simulink model "iterateddes"  (R2024b)
settings: Solver=VariableStepAuto  StartTime=0.0  StopTime=5  RelTol=1e-3
undefined symbols (not defined in the file or in its folder): entity, m, n, recordQueueTimeEng1, recordQueueTimeSrEng1, recordQueueTimeSrEng2, recordQueueTimeSrEng3, recordTotalTimeAdmin, recordTotalTimeInc, recordTotalTimeMaint, recordTotalTimeProj, recordTotalTimeReq
settings Model: Creator=enos9  LastModifiedBy=enos9
settings SolverCC: AlgebraicLoopSolver=TrustRegion
settings DataIOCC: SaveOutput=off  SaveTime=off
settings DebuggingCC: UnconnectedInputMsg=warning  UnconnectedOutputMsg=warning  UnconnectedLineMsg=warning  ArithmeticOperatorsInVariantConditions=warning
settings ModelReferenceCC: EnableRefExpFcnMdlSchedulingChecks=on
settings SFSimCC: SimUseLocalCustomCode=off  CustomCodeUndefinedFunction=UseInterfaceOnly
settings RTWCC: RTWUseLocalCustomCode=off  GPUComputeCapability=3.5
settings CodeAppCC: StateflowObjectComments=on

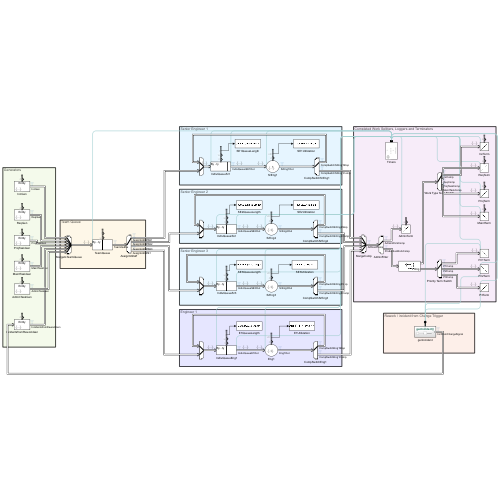
[thumbnail: Simulink's stored preview of the top-level diagram]
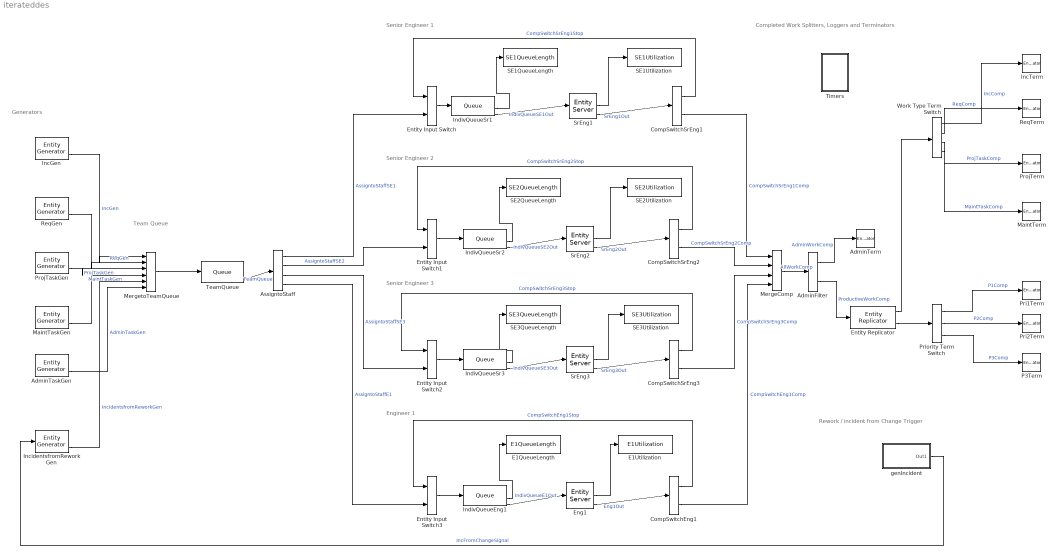
== system iterateddes ==
  note: Rework / incident from Change Trigger
  note: Completed Work Splitters, Loggers and Terminators
  note: Team Queue
  note: Senior Engineer 1
  note: Senior Engineer 2
  note: Senior Engineer 3
  note: Generators
  note: Engineer 1
  " IndivQueueEng1" : Queue  InputPortMessageModes=m  OutputPortMessageModes=n,n,n,m  Capacity=inf  QueueType=Priority  PrioritySource=Priority  EntryAction=entity.QueueTime = getStartTime();  ExitAction=recordQueueTimeEng1(entity.QueueTime)  NumberEntitiesInBlock=on  AverageWait=on  AverageQueueLength=on
      settings: OutputPortMap=o1,o2,o3,o5
  " IndivQueueSr3" : Queue  InputPortMessageModes=m  OutputPortMessageModes=n,n,n,m  Capacity=inf  QueueType=Priority  PrioritySource=Priority  EntryAction=entity.QueueTime = getStartTime();  ExitAction=recordQueueTimeSrEng3(entity.QueueTime)  NumberEntitiesInBlock=on  AverageWait=on  AverageQueueLength=on
      settings: OutputPortMap=o1,o2,o3,o5
  AdminFilter : EntityOutputSwitch  InputPortMessageModes=m  OutputPortMessageModes=m,m  SwitchingCriterion=From attribute  SwitchAttributeName=IsAdmin
  AdminTaskGen : EntityGenerator  OutputPortMessageModes=n,m  TimeSource=MATLAB action  IntergenerationTimeAction=dt = -.1*log(1-rand());  GenerateAction=|  AttributeName=Priority|ReqSkillLevel|ReqSkillType|ReqServiceTime|LeadTime|Urgency|RemWork|ServiceTime|AsignSkillLevel|Rework|WorkType|StartTime|QueueTime|ServiceStartTime|ServiceTimeAct|IsAdmin  AttributeInitialValue=0|3|0|.08|0|0|0|0|0|.005|5|1|0|1|.1|1  NumberEntitiesDeparted=on  EntityType=Structured  EntityTypeName=Entity
      | prnum = rand()                     %Priority
      | 
      | if prnum<0.6
      |     entity.Priority = 3;           %59 percent low priority
      | elseif prnum>0.995
      |     entity.Priority = 1;           %0.5 percent high priority
      | else
      |     entity.Priority = 2            %40 percent medium priority
      | end
      | 
      | pstnum = rand()                    %ReqSkillType
      | 
      | if pstnum<0.57                    
      |     entity.ReqSkillType = 2;       %56 percent team B (IDM)
      | elseif pstnum>0.89
      |     entity.ReqSkillType = 3;       %10 percent both
      | else
      |     entity.ReqSkillType = 1        %34 percent team A (O365)
      | end
      | 
      | %entity.ReqServiceTime = -.08*log(1-rand())       %ReqServiceTime
      settings: OutputPortMap=o0,o3
  AdminTerm : EntityTerminator  InputPortMessageModes=m  EntryAction=recordTotalTimeAdmin(entity.StartTime);  NumberEntitiesArrived=on
      settings: OutputPortMap=o0
  AssigntoStaff : EntityOutputSwitch  InputPortMessageModes=m  OutputPortMessageModes=m,m,m,m  NumberOutputPorts=4  SwitchingCriterion=Round robin  SwitchAttributeName=Attribute1
      settings: OutputPortMap=o0,o1,o2,o3
  CompSwitchEng1 : EntityOutputSwitch  InputPortMessageModes=m  OutputPortMessageModes=m,m  SwitchingCriterion=From attribute  SwitchAttributeName=RemWork
  CompSwitchSrEng1 : EntityOutputSwitch  InputPortMessageModes=m  OutputPortMessageModes=m,m  SwitchingCriterion=From attribute  SwitchAttributeName=RemWork
  CompSwitchSrEng2 : EntityOutputSwitch  InputPortMessageModes=m  OutputPortMessageModes=m,m  SwitchingCriterion=From attribute  SwitchAttributeName=RemWork
  CompSwitchSrEng3 : EntityOutputSwitch  InputPortMessageModes=m  OutputPortMessageModes=m,m  SwitchingCriterion=From attribute  SwitchAttributeName=RemWork
  E1QueueLength : ToWorkspace  VariableName=E1QueueLength  SaveFormat=Timeseries  SampleTime=-1
  E1Utilization : ToWorkspace  VariableName=E1Utilization  SaveFormat=Timeseries  SampleTime=-1
  Eng1 : EntityServer  InputPortMessageModes=m  OutputPortMessageModes=n,n,m  Capacity=1  ServiceTimeSource=Attribute  ServiceTimeAction=|  EntryAction=|  ServiceCompleteAction=|  NumberEntitiesDeparted=on  Utilization=on
      ServiceTimeAction=|
      | mean = .5;
      | dt = -mean*log(1-rand());
      EntryAction=|
      | AvailableTime = -(entity.ServiceTimeAct)*log(1-rand());
      | if entity.ReqServiceTime < AvailableTime
      |     entity.ServiceTime = -(entity.ReqServiceTime)*log(1-rand());
      | else
      |     entity.ServiceTime = AvailableTime
      | end
      | 
      | entity.ServiceStartTime = getStartTime()-entity.QueueTime;
      | 
      | entity.AsignSkillLevel = 2
      | 
      | skilvldiff = entity.AsignSkillLevel - entity.ReqSkillLevel
      | if skilvldiff == 2
      |     entity.ServiceTime = entity.ServiceTime*0.80
      |     entity.Rework = entity.Rework-0.002
      | elseif skilvldiff == 1
      |     entity.ServiceTime = entity.ServiceTime*0.90
      |     entity.Rework = entity.Rework-0.001
      | elseif skilvldiff == -1
      |     entity.ServiceTime = entity.ServiceTime*1.1
      |     entity.Rework = entity.Rework+0.0025
      | elseif skilvldiff == -2
      |     entity.ServiceTime = entity.ServiceTime*1.2
      |     entity.Rework = entity.Rework+0.005
      | end
      ServiceCompleteAction=|
      | svctimediff = entity.ReqServiceTime - entity.ServiceTime
      | 
      | if svctimediff > 0
      |     entity.RemWork = 1
      |     entity.ReqServiceTime = svctimediff * 1.1
      | else
      |     entity.RemWork = 2
      | end
      settings: OutputPortMap=o0,o5,o9
  Entity Input Switch : EntityInputSwitch  InputPortMessageModes=m,m  OutputPortMessageModes=m  SwitchingCriterion=Equiprobable
  Entity Input Switch1 : EntityInputSwitch  InputPortMessageModes=m,m  OutputPortMessageModes=m
  Entity Input Switch2 : EntityInputSwitch  InputPortMessageModes=m,m  OutputPortMessageModes=m
  Entity Input Switch3 : EntityInputSwitch  InputPortMessageModes=m,m  OutputPortMessageModes=m
  Entity Replicator : EntityReplicator  InputPortMessageModes=m  OutputPortMessageModes=m,m
  IncGen : EntityGenerator  Description=Incident Generator  OutputPortMessageModes=n,m  TimeSource=MATLAB action  IntergenerationTimeAction=dt = -0.2024906*log(1-rand());  GenerateAction=|  AttributeName=Priority|ReqSkillLevel|ReqSkillType|ReqServiceTime|LeadTime|Urgency|RemWork|ServiceTime|AsignSkillLevel|Rework|WorkType|StartTime|QueueTime|ServiceStartTime|ServiceTimeAct|IsAdmin  AttributeInitialValue=0|0|0|.08|0|0|0|0|0|.005|1|1|0|1|.1|2  NumberEntitiesDeparted=on  EntityType=Structured  EntityTypeName=Entity
      | prnum = rand()                     %Priority
      | 
      | if prnum<0.6
      |     entity.Priority = 3;           %59 percent low priority
      | elseif prnum>0.995
      |     entity.Priority = 1;           %0.5 percent high priority
      | else
      |     entity.Priority = 2            %40.5 percent medium priority
      | end
      | 
      | pslnum = rand()                    %ReqSkillLevel
      | 
      | if pslnum<0.76
      |     entity.ReqSkillLevel = 3;      %75 percent low skill
      | elseif pslnum>0.94
      |     entity.ReqSkillLevel = 1;      %5 percent high skill
      | else
      |     entity.ReqSkillLevel = 2       %20 percent medium skill
      | end
      | 
      | pstnum = rand()                    %ReqSkillType
      | 
      | if pstnum<0.57                    
      |     entity.ReqSkillType = 2;       %56 percent team B (IDM)
      | elseif pstnum>0.89
      |     entity.ReqSkillType = 3;       %10 percent both
      | else
      |     entity.ReqSkillType = 1        %34 percent team A (O365)
      | end
      settings: OutputPortMap=o0,o3
  IncTerm : EntityTerminator  InputPortMessageModes=m  EntryAction=recordTotalTimeInc(entity.StartTime);  NumberEntitiesArrived=on
      settings: OutputPortMap=o0
  IncidentsfromReworkGen : EntityGenerator  InputPortMessageModes=m  OutputPortMessageModes=n,m  GenerationMethod=Event-based  GenerateAction=|  AttributeName=Priority|ReqSkillLevel|ReqSkillType|ReqServiceTime|LeadTime|Urgency|RemWork|ServiceTime|AsignSkillLevel|Rework|WorkType|StartTime|QueueTime|ServiceStartTime|ServiceTimeAct|IsAdmin  AttributeInitialValue=0|0|0|.08|0|0|0|0|0|.005|1|1|0|1|.1|2  NumberEntitiesDeparted=on  EntityType=Structured  EntityTypeName=Entity
      | prnum = rand()                     %Priority
      | 
      | if prnum<0.6
      |     entity.Priority = 3;           %59 percent low priority
      | elseif prnum>0.995
      |     entity.Priority = 1;           %0.5 percent high priority
      | else
      |     entity.Priority = 2            %40 percent medium priority
      | end
      | 
      | pslnum = rand()                    %ReqSkillLevel
      | 
      | if pslnum<0.76
      |     entity.ReqSkillLevel = 3;      %75 percent low skill
      | elseif pslnum>0.94
      |     entity.ReqSkillLevel = 1;      %5 percent high skill
      | else
      |     entity.ReqSkillLevel = 2       %20 percent medium skill
      | end
      | 
      | pstnum = rand()                    %ReqSkillType
      | 
      | if pstnum<0.57                    
      |     entity.ReqSkillType = 2;       %56 percent team B (IDM)
      | elseif pstnum>0.89
      |     entity.ReqSkillType = 3;       %10 percent both
      | else
      |     entity.ReqSkillType = 1        %34 percent team A (O365)
      | end
      | 
      | %entity.ReqServiceTime = -.08*log(1-rand())       %ReqServiceTime
      settings: InputPortMap=u0  OutputPortMap=o0,o3
  IndivQueueSr1 : Queue  InputPortMessageModes=m  OutputPortMessageModes=n,n,n,m  Capacity=inf  QueueType=Priority  PrioritySource=Priority  EntryAction=entity.QueueTime = getStartTime();  ExitAction=recordQueueTimeSrEng1(entity.QueueTime)  NumberEntitiesInBlock=on  AverageWait=on  AverageQueueLength=on
      settings: OutputPortMap=o1,o2,o3,o5
  IndivQueueSr2 : Queue  InputPortMessageModes=m  OutputPortMessageModes=n,n,n,m  Capacity=inf  QueueType=Priority  PrioritySource=Priority  EntryAction=entity.QueueTime = getStartTime();  ExitAction=recordQueueTimeSrEng2(entity.QueueTime)  NumberEntitiesInBlock=on  AverageWait=on  AverageQueueLength=on
      settings: OutputPortMap=o1,o2,o3,o5
  MaintTaskGen : EntityGenerator  Description=Request Generator  OutputPortMessageModes=n,m  TimeSource=MATLAB action  IntergenerationTimeAction=dt = -.125*log(1-rand());  GenerateAction=|  AttributeName=Priority|ReqSkillLevel|ReqSkillType|ReqServiceTime|LeadTime|Urgency|RemWork|ServiceTime|AsignSkillLevel|Rework|WorkType|StartTime|QueueTime|ServiceStartTime|ServiceTimeAct|IsAdmin  AttributeInitialValue=0|0|0|.08|0|0|0|0|0|.005|4|1|0|1|.1|2  NumberEntitiesDeparted=on  EntityType=Structured  EntityTypeName=Entity
      | prnum = rand()                     %Priority
      | 
      | if prnum<0.6
      |     entity.Priority = 3;           %59 percent low priority
      | elseif prnum>0.995
      |     entity.Priority = 1;           %0.5 percent high priority
      | else
      |     entity.Priority = 2            %40 percent medium priority
      | end
      | 
      | pslnum = rand()                    %ReqSkillLevel
      | 
      | if pslnum<0.76
      |     entity.ReqSkillLevel = 3;      %75 percent low skill
      | elseif pslnum>0.94
      |     entity.ReqSkillLevel = 1;      %5 percent high skill
      | else
      |     entity.ReqSkillLevel = 2       %20 percent medium skill
      | end
      | 
      | pstnum = rand()                    %ReqSkillType
      | 
      | if pstnum<0.57                    
      |     entity.ReqSkillType = 2;       %56 percent team B (IDM)
      | elseif pstnum>0.89
      |     entity.ReqSkillType = 3;       %10 percent both
      | else
      |     entity.ReqSkillType = 1        %34 percent team A (O365)
      | end
      | 
      | %entity.ReqServiceTime = -.08*log(1-rand())       %ReqServiceTime
      settings: OutputPortMap=o0,o3
  MaintTerm : EntityTerminator  InputPortMessageModes=m  EntryAction=recordTotalTimeMaint(entity.StartTime);  NumberEntitiesArrived=on
      settings: OutputPortMap=o0
  MergeComp : EntityInputSwitch  InputPortMessageModes=m,m,m,m  OutputPortMessageModes=m  NumberInputPorts=4
      settings: InputPortMap=u1,u2,u3,u4
  MergetoTeamQueue : EntityInputSwitch  InputPortMessageModes=m,m,m,m,m,m  OutputPortMessageModes=m  NumberInputPorts=6
      settings: InputPortMap=u1,u2,u3,u4,u5,u6
  P3Term : EntityTerminator  InputPortMessageModes=m  EntryAction=|
      | recordTotalTimeP3(entity.StartTime);
      | 
      | rewnum = rand()
      | 
      | if rewnum < entity.Rework
      |     genIncident();
      |     
      | end
  Pri1Term : EntityTerminator  InputPortMessageModes=m  EntryAction=|
      | recordTotalTimeP1(entity.StartTime);
      | 
      | rewnum = rand()
      | 
      | if rewnum < entity.Rework
      |     genIncident();
      |     
      | end
  Pri2Term : EntityTerminator  InputPortMessageModes=m  EntryAction=|
      | recordTotalTimeP2(entity.StartTime);
      | 
      | rewnum = rand()
      | 
      | if rewnum < entity.Rework
      |     genIncident();
      |     
      | end
  Priority Term Switch : EntityOutputSwitch  InputPortMessageModes=m  OutputPortMessageModes=m,m,m  NumberOutputPorts=3  SwitchingCriterion=From attribute  SwitchAttributeName=Priority
      settings: OutputPortMap=o0,o1,o2
  ProjTaskGen : EntityGenerator  Description=Request Generator  OutputPortMessageModes=n,m  TimeSource=MATLAB action  IntergenerationTimeAction=dt = -.2*log(1-rand());  GenerateAction=|  AttributeName=Priority|ReqSkillLevel|ReqSkillType|ReqServiceTime|LeadTime|Urgency|RemWork|ServiceTime|AsignSkillLevel|Rework|WorkType|StartTime|QueueTime|ServiceStartTime|ServiceTimeAct|IsAdmin  AttributeInitialValue=0|0|0|.08|0|0|0|0|0|.005|3|1|0|1|.1|2  NumberEntitiesDeparted=on  EntityType=Structured  EntityTypeName=Entity
      | prnum = rand()                     %Priority
      | 
      | if prnum<0.6
      |     entity.Priority = 3;           %59 percent low priority
      | elseif prnum>0.995
      |     entity.Priority = 1;           %0.5 percent high priority
      | else
      |     entity.Priority = 2            %40 percent medium priority
      | end
      | 
      | pslnum = rand()                    %ReqSkillLevel
      | 
      | if pslnum<0.76
      |     entity.ReqSkillLevel = 3;      %75 percent low skill
      | elseif pslnum>0.94
      |     entity.ReqSkillLevel = 1;      %5 percent high skill
      | else
      |     entity.ReqSkillLevel = 2       %20 percent medium skill
      | end
      | 
      | pstnum = rand()                    %ReqSkillType
      | 
      | if pstnum<0.57                    
      |     entity.ReqSkillType = 2;       %56 percent team B (IDM)
      | elseif pstnum>0.89
      |     entity.ReqSkillType = 3;       %10 percent both
      | else
      |     entity.ReqSkillType = 1        %34 percent team A (O365)
      | end
      | 
      | %entity.ReqServiceTime = -.08*log(1-rand())       %ReqServiceTime
      settings: OutputPortMap=o0,o3
  ProjTerm : EntityTerminator  InputPortMessageModes=m  EntryAction=recordTotalTimeProj(entity.StartTime);  NumberEntitiesArrived=on
      settings: OutputPortMap=o0
  ReqGen : EntityGenerator  Description=Request Generator  OutputPortMessageModes=n,m  TimeSource=MATLAB action  IntergenerationTimeAction=dt = -0.0930726*log(1-rand());  GenerateAction=|  AttributeName=Priority|ReqSkillLevel|ReqSkillType|ReqServiceTime|LeadTime|Urgency|RemWork|ServiceTime|AsignSkillLevel|Rework|WorkType|StartTime|QueueTime|ServiceStartTime|ServiceTimeAct|IsAdmin  AttributeInitialValue=0|0|0|.08|0|0|0|0|0|.005|2|1|0|1|.1|2  NumberEntitiesDeparted=on  EntityType=Structured  EntityTypeName=Entity
      | prnum = rand()                     %Priority
      | 
      | if prnum<0.6
      |     entity.Priority = 3;           %59 percent low priority
      | elseif prnum>0.995
      |     entity.Priority = 1;           %0.5 percent high priority
      | else
      |     entity.Priority = 2            %40 percent medium priority
      | end
      | 
      | pslnum = rand()                    %ReqSkillLevel
      | 
      | if pslnum<0.76
      |     entity.ReqSkillLevel = 3;      %75 percent low skill
      | elseif pslnum>0.94
      |     entity.ReqSkillLevel = 1;      %5 percent high skill
      | else
      |     entity.ReqSkillLevel = 2       %20 percent medium skill
      | end
      | 
      | pstnum = rand()                    %ReqSkillType
      | 
      | if pstnum<0.57                    
      |     entity.ReqSkillType = 2;       %56 percent team B (IDM)
      | elseif pstnum>0.89
      |     entity.ReqSkillType = 3;       %10 percent both
      | else
      |     entity.ReqSkillType = 1        %34 percent team A (O365)
      | end
      | 
      | %entity.ReqServiceTime = -.08*log(1-rand())       %ReqServiceTime
      settings: OutputPortMap=o0,o3
  ReqTerm : EntityTerminator  InputPortMessageModes=m  EntryAction=recordTotalTimeReq(entity.StartTime);  NumberEntitiesArrived=on
      settings: OutputPortMap=o0
  SE1QueueLength : ToWorkspace  VariableName=SE1QueueLength  SaveFormat=Timeseries  SampleTime=-1
  SE1Utilization : ToWorkspace  VariableName=SE1Utilization  SaveFormat=Timeseries  SampleTime=-1
  SE2QueueLength : ToWorkspace  VariableName=SE2QueueLength  SaveFormat=Timeseries  SampleTime=-1
  SE2Utilization : ToWorkspace  VariableName=SE2Utilization  SaveFormat=Timeseries  SampleTime=-1
  SE3QueueLength : ToWorkspace  VariableName=SE3QueueLength  SaveFormat=Timeseries  SampleTime=-1
  SE3Utilization : ToWorkspace  VariableName=SE3Utilization  SaveFormat=Timeseries  SampleTime=-1
  SrEng1 : EntityServer  InputPortMessageModes=m  OutputPortMessageModes=n,n,m  Capacity=1  ServiceTimeSource=Attribute  ServiceTimeAction=|  EntryAction=|  ServiceCompleteAction=|  NumberEntitiesDeparted=on  Utilization=on
      ServiceTimeAction=|
      | mean = .3;
      | dt = -mean*log(1-rand());
      EntryAction=|
      | AvailableTime = -(entity.ServiceTimeAct)*log(1-rand());
      | if entity.ReqServiceTime < AvailableTime
      |     entity.ServiceTime = -(entity.ReqServiceTime)*log(1-rand());
      | else
      |     entity.ServiceTime = AvailableTime
      | end
      | 
      | entity.ServiceStartTime = getStartTime()-entity.QueueTime;
      | 
      | entity.AsignSkillLevel = 1
      | 
      | skilvldiff = entity.AsignSkillLevel - entity.ReqSkillLevel
      | if skilvldiff == 2
      |     entity.ServiceTime = entity.ServiceTime*0.80
      |     entity.Rework = entity.Rework-0.002
      | elseif skilvldiff == 1
      |     entity.ServiceTime = entity.ServiceTime*0.90
      |     entity.Rework = entity.Rework-0.001
      | elseif skilvldiff == -1
      |     entity.ServiceTime = entity.ServiceTime*1.1
      |     entity.Rework = entity.Rework+0.0025
      | elseif skilvldiff == -2
      |     entity.ServiceTime = entity.ServiceTime*1.2
      |     entity.Rework = entity.Rework+0.005
      | end
      ServiceCompleteAction=|
      | svctimediff = entity.ReqServiceTime - entity.ServiceTime
      | 
      | if svctimediff > 0
      |     entity.RemWork = 1
      |     entity.ReqServiceTime = svctimediff * 1.1
      | else
      |     entity.RemWork = 2
      | end
      settings: OutputPortMap=o0,o5,o9
  SrEng2 : EntityServer  InputPortMessageModes=m  OutputPortMessageModes=n,n,m  Capacity=1  ServiceTimeSource=Attribute  ServiceTimeAction=|  EntryAction=|  ServiceCompleteAction=|  NumberEntitiesDeparted=on  Utilization=on
      ServiceTimeAction=|
      | mean = .3;
      | dt = -mean*log(1-rand());
      EntryAction=|
      | AvailableTime = -(entity.ServiceTimeAct)*log(1-rand());
      | if entity.ReqServiceTime < AvailableTime
      |     entity.ServiceTime = -(entity.ReqServiceTime)*log(1-rand());
      | else
      |     entity.ServiceTime = AvailableTime
      | end
      | 
      | entity.ServiceStartTime = getStartTime()-entity.QueueTime;
      | 
      | entity.AsignSkillLevel = 1
      | 
      | skilvldiff = entity.AsignSkillLevel - entity.ReqSkillLevel
      | if skilvldiff == 2
      |     entity.ServiceTime = entity.ServiceTime*0.80
      |     entity.Rework = entity.Rework-0.002
      | elseif skilvldiff == 1
      |     entity.ServiceTime = entity.ServiceTime*0.90
      |     entity.Rework = entity.Rework-0.001
      | elseif skilvldiff == -1
      |     entity.ServiceTime = entity.ServiceTime*1.1
      |     entity.Rework = entity.Rework+0.0025
      | elseif skilvldiff == -2
      |     entity.ServiceTime = entity.ServiceTime*1.2
      |     entity.Rework = entity.Rework+0.005
      | end
      ServiceCompleteAction=|
      | svctimediff = entity.ReqServiceTime - entity.ServiceTime
      | 
      | if svctimediff > 0
      |     entity.RemWork = 1
      |     entity.ReqServiceTime = svctimediff * 1.1
      | else
      |     entity.RemWork = 2
      | end
      settings: OutputPortMap=o0,o5,o9
  SrEng3 : EntityServer  InputPortMessageModes=m  OutputPortMessageModes=n,n,m  Capacity=1  ServiceTimeSource=Attribute  ServiceTimeAction=|  EntryAction=|  ServiceCompleteAction=|  NumberEntitiesDeparted=on  Utilization=on
      ServiceTimeAction=|
      | mean = .3;
      | dt = -mean*log(1-rand());
      EntryAction=|
      | AvailableTime = -(entity.ServiceTimeAct)*log(1-rand());
      | if entity.ReqServiceTime < AvailableTime
      |     entity.ServiceTime = -(entity.ReqServiceTime)*log(1-rand());
      | else
      |     entity.ServiceTime = AvailableTime
      | end
      | 
      | entity.ServiceStartTime = getStartTime()-entity.QueueTime;
      | 
      | entity.AsignSkillLevel = 1
      | 
      | skilvldiff = entity.AsignSkillLevel - entity.ReqSkillLevel
      | if skilvldiff == 2
      |     entity.ServiceTime = entity.ServiceTime*0.80
      |     entity.Rework = entity.Rework-0.002
      | elseif skilvldiff == 1
      |     entity.ServiceTime = entity.ServiceTime*0.90
      |     entity.Rework = entity.Rework-0.001
      | elseif skilvldiff == -1
      |     entity.ServiceTime = entity.ServiceTime*1.1
      |     entity.Rework = entity.Rework+0.0025
      | elseif skilvldiff == -2
      |     entity.ServiceTime = entity.ServiceTime*1.2
      |     entity.Rework = entity.Rework+0.005
      | end
      ServiceCompleteAction=|
      | svctimediff = entity.ReqServiceTime - entity.ServiceTime
      | 
      | if svctimediff > 0
      |     entity.RemWork = 1
      |     entity.ReqServiceTime = svctimediff * 1.1
      | else
      |     entity.RemWork = 2
      | end
      settings: OutputPortMap=o0,o5,o9
  TeamQueue : Queue  Description=Team Queue  InputPortMessageModes=m  OutputPortMessageModes=n,n,m  Capacity=inf  QueueType=Priority  PrioritySource=Priority  EntryAction=entity.StartTime = getStartTime();  AverageWait=on  AverageQueueLength=on
      settings: OutputPortMap=o2,o3,o5
  Timers : Subsystem
  Work Type Term Switch : EntityOutputSwitch  InputPortMessageModes=m  OutputPortMessageModes=m,m,m,m  NumberOutputPorts=4  SwitchingCriterion=From attribute  SwitchAttributeName=WorkType
      settings: OutputPortMap=o0,o1,o2,o3
  genIncident : Subsystem  TreatAsAtomicUnit=on
  wires:
  IndivQueueSr1/4 -> SrEng1/1  "IndivQueueSE1Out"
  SrEng1/3 -> CompSwitchSrEng1/1  "SrEng1Out"
  IncGen/2 -> MergetoTeamQueue/1  "IncGen"
  ReqGen/2 -> MergetoTeamQueue/2  "ReqGen"
  TeamQueue/3 -> AssigntoStaff/1  "TeamQueue"
  SrEng2/3 -> CompSwitchSrEng2/1  "SrEng2Out"
  IndivQueueSr2/4 -> SrEng2/1  "IndivQueueSE2Out"
  AssigntoStaff/1 -> Entity Input Switch/2  "AssigntoStaffSE1"
  AssigntoStaff/2 -> Entity Input Switch1/2  "AssigntoStaffSE2"
  SrEng3/3 -> CompSwitchSrEng3/1  "SrEng3Out"
  " IndivQueueSr3"/4 -> SrEng3/1  "IndivQueueSE3Out"
  AssigntoStaff/3 -> Entity Input Switch2/2  "AssigntoStaffSE3"
  Eng1/3 -> CompSwitchEng1/1  "Eng1Out"
  " IndivQueueEng1"/4 -> Eng1/1  "IndivQueueE1Out"
  AssigntoStaff/4 -> Entity Input Switch3/2  "AssigntoStaffE1"
  SrEng1/2 -> SE1Utilization/1
  SrEng2/2 -> SE2Utilization/1
  SrEng3/2 -> SE3Utilization/1
  Eng1/2 -> E1Utilization/1
  ProjTaskGen/2 -> MergetoTeamQueue/3  "ProjTaskGen"
  MergeComp/1 -> AdminFilter/1  "AllWorkComp"
  MaintTaskGen/2 -> MergetoTeamQueue/4  "MaintTaskGen"
  MergetoTeamQueue/1 -> TeamQueue/1
  CompSwitchSrEng1/1 -> Entity Input Switch/1  "CompSwitchSrEng1Stop"
  Entity Input Switch/1 -> IndivQueueSr1/1
  CompSwitchSrEng1/2 -> MergeComp/1  "CompSwitchSrEng1Comp"
  CompSwitchSrEng2/2 -> MergeComp/2  "CompSwitchSrEng2Comp"
  CompSwitchSrEng2/1 -> Entity Input Switch1/1  "CompSwitchSrEng2Stop"
  Entity Input Switch1/1 -> IndivQueueSr2/1
  CompSwitchSrEng3/1 -> Entity Input Switch2/1  "CompSwitchSrEng3Stop"
  CompSwitchSrEng3/2 -> MergeComp/3  "CompSwitchSrEng3Comp"
  Entity Input Switch2/1 -> " IndivQueueSr3"/1
  CompSwitchEng1/1 -> Entity Input Switch3/1  "CompSwitchEng1Stop"
  Entity Input Switch3/1 -> " IndivQueueEng1"/1
  CompSwitchEng1/2 -> MergeComp/4  "CompSwitchEng1Comp"
  IncidentsfromReworkGen/2 -> MergetoTeamQueue/5  "IncidentsfromReworkGen"
  genIncident/1(Out1) -> IncidentsfromReworkGen/1  "IncFromChangeSignal"
  Priority Term Switch/1 -> Pri1Term/1  "P1Comp"
  Priority Term Switch/2 -> Pri2Term/1  "P2Comp"
  Priority Term Switch/3 -> P3Term/1  "P3Comp"
  Entity Replicator/2 -> Priority Term Switch/1
  Entity Replicator/1 -> Work Type Term Switch/1
  Work Type Term Switch/1 -> IncTerm/1  "IncComp"
  Work Type Term Switch/2 -> ReqTerm/1  "ReqComp"
  Work Type Term Switch/3 -> ProjTerm/1  "ProjTaskComp"
  Work Type Term Switch/4 -> MaintTerm/1  "MaintTaskComp"
  IndivQueueSr1/3 -> SE1QueueLength/1
  IndivQueueSr2/3 -> SE2QueueLength/1
  " IndivQueueSr3"/3 -> SE3QueueLength/1
  " IndivQueueEng1"/3 -> E1QueueLength/1
  AdminTaskGen/2 -> MergetoTeamQueue/6  "AdminTaskGen"
  AdminFilter/2 -> Entity Replicator/1  "ProductiveWorkComp"
  AdminFilter/1 -> AdminTerm/1  "AdminWorkComp"

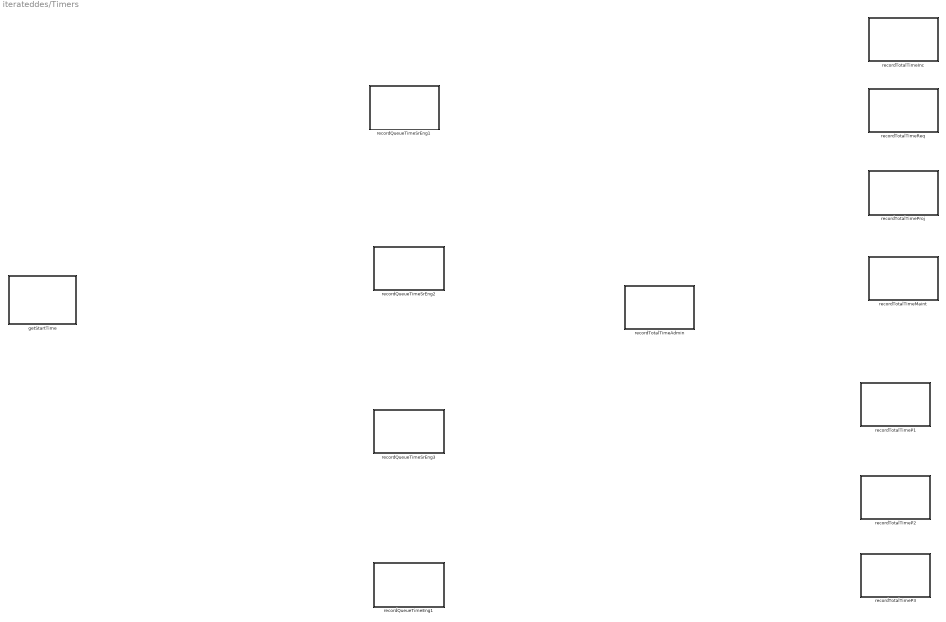
== system iterateddes/Timers ==
  getStartTime : Subsystem  TreatAsAtomicUnit=on
  recordQueueTimeEng1 : Subsystem  TreatAsAtomicUnit=on
  recordQueueTimeSrEng1 : Subsystem  TreatAsAtomicUnit=on
  recordQueueTimeSrEng2 : Subsystem  TreatAsAtomicUnit=on
  recordQueueTimeSrEng3 : Subsystem  TreatAsAtomicUnit=on
  recordTotalTimeAdmin : Subsystem  TreatAsAtomicUnit=on
  recordTotalTimeInc : Subsystem  TreatAsAtomicUnit=on
  recordTotalTimeMaint : Subsystem  TreatAsAtomicUnit=on
  recordTotalTimeP1 : Subsystem  TreatAsAtomicUnit=on
  recordTotalTimeP2 : Subsystem  TreatAsAtomicUnit=on
  recordTotalTimeP3 : Subsystem  TreatAsAtomicUnit=on
  recordTotalTimeProj : Subsystem  TreatAsAtomicUnit=on
  recordTotalTimeReq : Subsystem  TreatAsAtomicUnit=on

== system iterateddes/genIncident ==
  genIncident : TriggerPort  TriggerType=function-call  IsSimulinkFunction=on  FunctionName=genIncident  FunctionVisibility=scoped  VariantControl=(inherit)
  Constant : Constant
  Message Send : Send  OutputPortMessageModes=m
  Out1 : Outport
  wires:
  Constant/1 -> Message Send/1
  Message Send/1 -> Out1/1

== system iterateddes/Timers/getStartTime ==
  getStartTime : TriggerPort  TriggerType=function-call  IsSimulinkFunction=on  FunctionName=getStartTime  VariantControl=(inherit)
  Digital Clock : DigitalClock  SampleTime=-1
  t : ArgOut  DisableCoverage=on  ArgumentName=t
  wires:
  Digital Clock/1 -> t/1

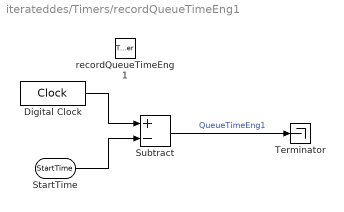
== system iterateddes/Timers/recordQueueTimeEng1 ==
  recordQueueTimeEng1 : TriggerPort  TriggerType=function-call  IsSimulinkFunction=on  FunctionName=recordQueueTimeEng1  VariantControl=(inherit)
  Digital Clock : DigitalClock  SampleTime=-1
  Subtract : Sum  Inputs=+-
  Terminator : Terminator
  StartTime : ArgIn  DisableCoverage=on  ArgumentName=StartTime
  wires:
  StartTime/1 -> Subtract/2
  Digital Clock/1 -> Subtract/1
  Subtract/1 -> Terminator/1  "QueueTimeEng1"

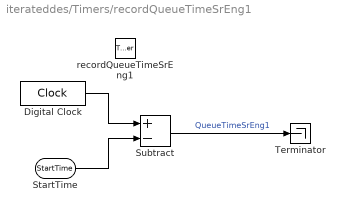
== system iterateddes/Timers/recordQueueTimeSrEng1 ==
  recordQueueTimeSrEng1 : TriggerPort  TriggerType=function-call  IsSimulinkFunction=on  FunctionName=recordQueueTimeSrEng1  VariantControl=(inherit)
  Digital Clock : DigitalClock  SampleTime=-1
  Subtract : Sum  Inputs=+-
  Terminator : Terminator
  StartTime : ArgIn  DisableCoverage=on  ArgumentName=StartTime
  wires:
  StartTime/1 -> Subtract/2
  Digital Clock/1 -> Subtract/1
  Subtract/1 -> Terminator/1  "QueueTimeSrEng1"

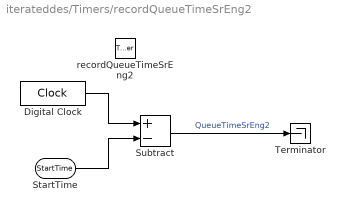
== system iterateddes/Timers/recordQueueTimeSrEng2 ==
  recordQueueTimeSrEng2 : TriggerPort  TriggerType=function-call  IsSimulinkFunction=on  FunctionName=recordQueueTimeSrEng2  VariantControl=(inherit)
  Digital Clock : DigitalClock  SampleTime=-1
  Subtract : Sum  Inputs=+-
  Terminator : Terminator
  StartTime : ArgIn  DisableCoverage=on  ArgumentName=StartTime
  wires:
  StartTime/1 -> Subtract/2
  Digital Clock/1 -> Subtract/1
  Subtract/1 -> Terminator/1  "QueueTimeSrEng2"

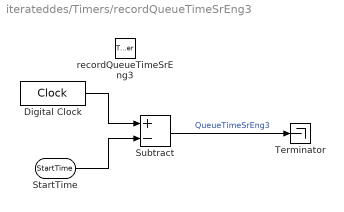
== system iterateddes/Timers/recordQueueTimeSrEng3 ==
  recordQueueTimeSrEng3 : TriggerPort  TriggerType=function-call  IsSimulinkFunction=on  FunctionName=recordQueueTimeSrEng3  VariantControl=(inherit)
  Digital Clock : DigitalClock  SampleTime=-1
  Subtract : Sum  Inputs=+-
  Terminator : Terminator
  StartTime : ArgIn  DisableCoverage=on  ArgumentName=StartTime
  wires:
  StartTime/1 -> Subtract/2
  Digital Clock/1 -> Subtract/1
  Subtract/1 -> Terminator/1  "QueueTimeSrEng3"

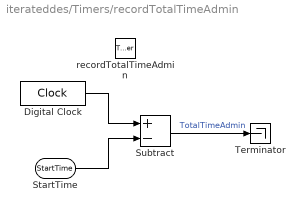
== system iterateddes/Timers/recordTotalTimeAdmin ==
  recordTotalTimeAdmin : TriggerPort  TriggerType=function-call  IsSimulinkFunction=on  FunctionName=recordTotalTimeAdmin  VariantControl=(inherit)
  Digital Clock : DigitalClock  SampleTime=-1
  Subtract : Sum  Inputs=+-
  Terminator : Terminator
  StartTime : ArgIn  DisableCoverage=on  ArgumentName=StartTime
  wires:
  StartTime/1 -> Subtract/2
  Digital Clock/1 -> Subtract/1
  Subtract/1 -> Terminator/1  "TotalTimeAdmin"

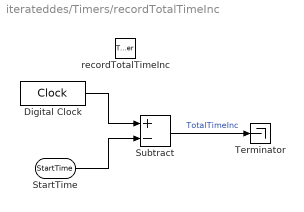
== system iterateddes/Timers/recordTotalTimeInc ==
  recordTotalTimeInc : TriggerPort  TriggerType=function-call  IsSimulinkFunction=on  FunctionName=recordTotalTimeInc  VariantControl=(inherit)
  Digital Clock : DigitalClock  SampleTime=-1
  Subtract : Sum  Inputs=+-
  Terminator : Terminator
  StartTime : ArgIn  DisableCoverage=on  ArgumentName=StartTime
  wires:
  StartTime/1 -> Subtract/2
  Digital Clock/1 -> Subtract/1
  Subtract/1 -> Terminator/1  "TotalTimeInc"

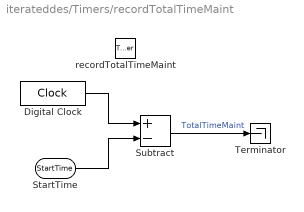
== system iterateddes/Timers/recordTotalTimeMaint ==
  recordTotalTimeMaint : TriggerPort  TriggerType=function-call  IsSimulinkFunction=on  FunctionName=recordTotalTimeMaint  VariantControl=(inherit)
  Digital Clock : DigitalClock  SampleTime=-1
  Subtract : Sum  Inputs=+-
  Terminator : Terminator
  StartTime : ArgIn  DisableCoverage=on  ArgumentName=StartTime
  wires:
  StartTime/1 -> Subtract/2
  Digital Clock/1 -> Subtract/1
  Subtract/1 -> Terminator/1  "TotalTimeMaint"

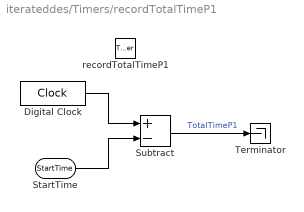
== system iterateddes/Timers/recordTotalTimeP1 ==
  recordTotalTimeP1 : TriggerPort  TriggerType=function-call  IsSimulinkFunction=on  FunctionName=recordTotalTimeP1  VariantControl=(inherit)
  Digital Clock : DigitalClock  SampleTime=-1
  Subtract : Sum  Inputs=+-
  Terminator : Terminator
  StartTime : ArgIn  DisableCoverage=on  ArgumentName=StartTime
  wires:
  StartTime/1 -> Subtract/2
  Digital Clock/1 -> Subtract/1
  Subtract/1 -> Terminator/1  "TotalTimeP1"

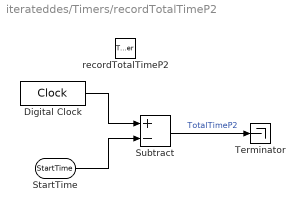
== system iterateddes/Timers/recordTotalTimeP2 ==
  recordTotalTimeP2 : TriggerPort  TriggerType=function-call  IsSimulinkFunction=on  FunctionName=recordTotalTimeP2  VariantControl=(inherit)
  Digital Clock : DigitalClock  SampleTime=-1
  Subtract : Sum  Inputs=+-
  Terminator : Terminator
  StartTime : ArgIn  DisableCoverage=on  ArgumentName=StartTime
  wires:
  StartTime/1 -> Subtract/2
  Digital Clock/1 -> Subtract/1
  Subtract/1 -> Terminator/1  "TotalTimeP2"

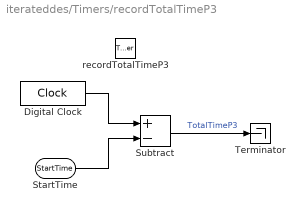
== system iterateddes/Timers/recordTotalTimeP3 ==
  recordTotalTimeP3 : TriggerPort  TriggerType=function-call  IsSimulinkFunction=on  FunctionName=recordTotalTimeP3  VariantControl=(inherit)
  Digital Clock : DigitalClock  SampleTime=-1
  Subtract : Sum  Inputs=+-
  Terminator : Terminator
  StartTime : ArgIn  DisableCoverage=on  ArgumentName=StartTime
  wires:
  StartTime/1 -> Subtract/2
  Digital Clock/1 -> Subtract/1
  Subtract/1 -> Terminator/1  "TotalTimeP3"

== system iterateddes/Timers/recordTotalTimeProj ==
  recordTotalTimeProj : TriggerPort  TriggerType=function-call  IsSimulinkFunction=on  FunctionName=recordTotalTimeProj  VariantControl=(inherit)
  Digital Clock : DigitalClock  SampleTime=-1
  Subtract : Sum  Inputs=+-
  Terminator : Terminator
  StartTime : ArgIn  DisableCoverage=on  ArgumentName=StartTime
  wires:
  StartTime/1 -> Subtract/2
  Digital Clock/1 -> Subtract/1
  Subtract/1 -> Terminator/1  "TotalTimeProj"

== system iterateddes/Timers/recordTotalTimeReq ==
  recordTotalTimeReq : TriggerPort  TriggerType=function-call  IsSimulinkFunction=on  FunctionName=recordTotalTimeReq  VariantControl=(inherit)
  Digital Clock : DigitalClock  SampleTime=-1
  Subtract : Sum  Inputs=+-
  Terminator : Terminator
  StartTime : ArgIn  DisableCoverage=on  ArgumentName=StartTime
  wires:
  StartTime/1 -> Subtract/2
  Digital Clock/1 -> Subtract/1
  Subtract/1 -> Terminator/1  "TotalTimeReq"
